simulink model "ErrLmp_DD"  (R2016b)
settings: configuration reference "CodeGenConfigSet" (kept outside this file)
values from neighbouring files (symbols this model uses):
  ErrLmp_stPsDiaDisbl_C = Calibration.Parameter    [init_ErrLmp_DD.m]
  ErrLmp_stPsDisbl_C = Calibration.Parameter    [init_ErrLmp_DD.m]
  SigTst_stErrLmp_C = Calibration.Parameter    [init_ErrLmp_DD.m]
  SigTst_swtErrLmp_C = Calibration.Parameter    [init_ErrLmp_DD.m]
undefined symbols (not defined in the file or in its folder): Switch_conv
libraries: simulink x4
settings Model: Creator=lenovo  LastModifiedBy=liutao
settings ConfigSetRef: SourceLocation=Base Workspace

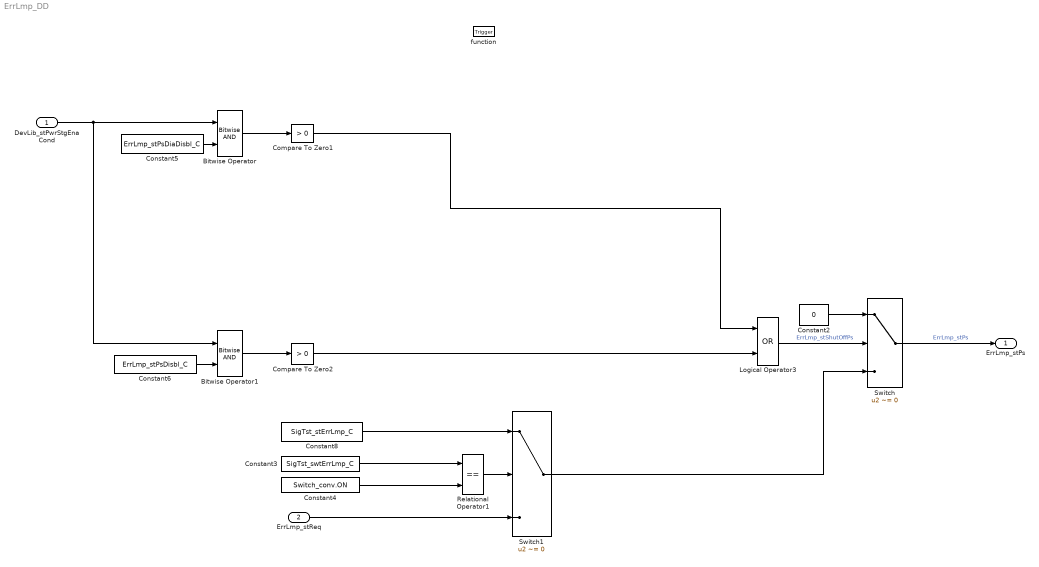
== system ErrLmp_DD ==
  DevLib_stPwrStgEnaCond : Inport  Description=Control unit status relevant to power stage deactivation/error diagnosis  OutMin=0  OutMax=65535  OutDataTypeStr=State_uint16
  ErrLmp_stReq : Inport  Description=Error request status  Port=2  OutMin=0  OutMax=1  OutDataTypeStr=boolean
  function : TriggerPort  TriggerType=function-call  VariantControl=Variant
  Bitwise Operator : simulink/Logic and Bit Operations/Bitwise Operator  logicop=AND  UseBitMask=off  NumInputPorts=2  BitMask=bin2dec('11011001')  BitMaskRealWorld=Stored Integer
  Bitwise Operator1 : simulink/Logic and Bit Operations/Bitwise Operator  logicop=AND  UseBitMask=off  NumInputPorts=2  BitMask=bin2dec('11011001')  BitMaskRealWorld=Stored Integer
  Compare To Zero1 : simulink/Logic and Bit Operations/Compare To Zero  relop=>  OutDataTypeStr=uint8
  Compare To Zero2 : simulink/Logic and Bit Operations/Compare To Zero  relop=>  OutDataTypeStr=boolean
  Constant2 : Constant  Value=0  OutDataTypeStr=boolean  SampleTime=-1
  Constant3 : Constant  Value=SigTst_swtErrLmp_C
  Constant4 : Constant  Value=Switch_conv.ON
  Constant5 : Constant  Value=ErrLmp_stPsDiaDisbl_C
  Constant6 : Constant  Value=ErrLmp_stPsDisbl_C
  Constant8 : Constant  Value=SigTst_stErrLmp_C
  Logical Operator3 : Logic  Operator=OR  AllPortsSameDT=off  OutDataTypeStr=boolean
  Relational Operator1 : RelationalOperator  Operator===  OutDataTypeStr=boolean  RndMeth=Nearest
  Switch : Switch  Criteria=u2 ~= 0  SaturateOnIntegerOverflow=on  InputSameDT=on
  Switch1 : Switch  Criteria=u2 ~= 0  SaturateOnIntegerOverflow=on  InputSameDT=on
  ErrLmp_stPs : Outport  Description=Digital output to the actuator after diagnosis  OutMin=0  OutMax=1  OutDataTypeStr=boolean
  wires:
  DevLib_stPwrStgEnaCond/1 -> Bitwise Operator/1, Bitwise Operator1/1
  Constant8/1 -> Switch1/1
  ErrLmp_stReq/1 -> Switch1/3
  Relational Operator1/1 -> Switch1/2
  Constant3/1 -> Relational Operator1/1
  Constant4/1 -> Relational Operator1/2
  Compare To Zero1/1 -> Logical Operator3/1
  Bitwise Operator/1 -> Compare To Zero1/1
  Constant5/1 -> Bitwise Operator/2
  Compare To Zero2/1 -> Logical Operator3/2
  Logical Operator3/1 -> Switch/2  "ErrLmp_stShutOffPs"
  Switch1/1 -> Switch/3
  Bitwise Operator1/1 -> Compare To Zero2/1
  Constant2/1 -> Switch/1
  Constant6/1 -> Bitwise Operator1/2
  Switch/1 -> ErrLmp_stPs/1  "ErrLmp_stPs"
